simulink model "AAIStateflow"  (R2020a)
settings: Solver=FixedStepAuto  StartTime=0.0  StopTime=10.0  FixedStep=1e-3  RelTol=1e-3  EnableMultiTasking=on
settings Model: ExtModeTrigDuration=5  Creator=liams  LastModifiedBy=liams
settings OptimizationCC: EnhancedBackFolding=on  PassReuseOutputArgsAs=Individual arguments  ZeroExternalMemoryAtStartup=off  ZeroInternalMemoryAtStartup=off  MaxStackSize=64  OptimizeBlockOrder=speed  DifferentSizesBufferReuse=on  OptimizationCustomize=off  EfficientTunableParamExpr=on
settings DebuggingCC: ParameterTunabilityLossMsg=error
settings HardwareCC: ProdBitPerPointer=32  ProdBitPerSizeT=32  ProdBitPerPtrDiffT=32  ProdLargestAtomicInteger=Long  ProdLargestAtomicFloat=Double  ProdWordSize=32  ProdHWDeviceType=ARM Compatible->ARM Cortex
settings SFSimCC: MATLABDynamicMemAlloc=off
settings RTWCC: SystemTargetFile=ert.tlc  HardwareBoard=NXP FRDM-K64F  TemplateMakefile=ert_default_tmf  Toolchain=GNU Tools for ARM Embedded Processors
settings CodeAppCC: ForceParamTrailComments=on  IgnoreCustomStorageClasses=off  OperatorAnnotations=on  SimulinkDataObjDesc=on  SFDataObjDesc=on  InsertBlockDesc=on

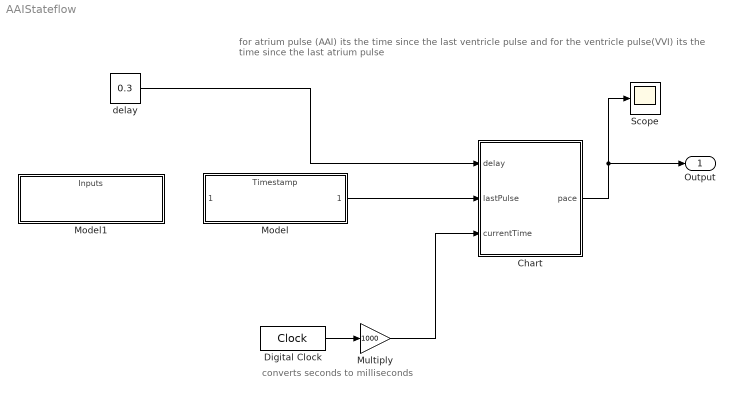
== system AAIStateflow ==
  note: converts seconds to milliseconds
  note: for atrium pulse (AAI) its the time since the last ventricle pulse and for the ventricle pulse(VVI) its the time since the last atrium pulse
  Chart : Stateflow chart  TreatAsAtomicUnit=on
  Digital Clock : DigitalClock
  Model : ModelReference  ModelNameDialog=Timestamp.slx  SimulationMode=Normal  ModelReferenceVersion=1.1
  Model1 : ModelReference  ModelNameDialog=Inputs.slx  SimulationMode=Normal  ModelReferenceVersion=1.9
  Multiply : Gain  Gain=1000
  Scope : Scope
  delay : Constant  Value=0.3
  Output : Outport
  wires:
  Chart/1(pace) -> Scope/1, Output/1
  delay/1 -> Chart/1(delay)
  Digital Clock/1 -> Multiply/1
  Multiply/1 -> Chart/3(currentTime)
  Model/1 -> Chart/2(lastPulse)

== stateflow chart AAIStateflow/Chart ==
  note: we will need it to pace if after a set delay the ventricle/atrium doesn't pump then the pacing will need to kick in
      | and pace for it
  state Pacing_Off
    entry:
    pace=false
  state Pacing_On
    entry:
    pace=true;
  note: t being the time since the last atrium/ventricle pulse
      | x being the time of the delay (x will need to be changed in the symbols panels because there is a
      | placeholder value there right now)
  (default) -> Pacing_Off
  Pacing_Off -> Pacing_On : [(currentTime-lastPulse)>delay]
  Pacing_On -> Pacing_Off : [true]
  data: pace output; delay input double =0.3; lastPulse input; currentTime input
